simulink model "RBCM_Model"  (R2024b)
settings: Solver=FixedStepAuto  StartTime=0.0  StopTime=10.0  RelTol=1e-3
PreLoadFcn:
  | % NXP_MBDT_S32K3 callback: DO NOT REMOVE
  | mbd_s32k3.common.nxp.model_callbacks.preLoadFcn();
PostLoadFcn:
  | % NXP_MBDT_S32K3 callback: DO NOT REMOVE
  | mbd_s32k3.common.nxp.model_callbacks.postLoadFcn();
InitFcn:
  | % NXP_MBDT_S32K3 callback: DO NOT REMOVE
  | mbd_s32k3.common.nxp.model_callbacks.initFcn();
undefined symbols (not defined in the file or in its folder): AccuFanPwr_hHsd3ch2, BspdPwr_lHsd1ch2, BuzzerPwr_lHsd3ch3, DevicePwr_12v_lHsd1ch1, DevicePwr_hHsd1ch2, DrsPwr_8v_lHsd3ch1, hHsd_Diagnose_AdcBuffer, ILPwr_hHsd1ch1, lHsd_Diagnose_AdcBuffer, LoggerPwr_lHsd1ch3, PumpFan1_hHsd4ch1, PumpFan2_hHsd4ch2, PumpPwr_hHsd3ch1, RGBLED0state, TaillightPwr_lHsd3ch4, TempSensorPwr_lHsd1ch4
libraries: mbd_s32k3_io_library x127, simulink x48, canmsglib x8, mbd_s32k3_communication_library x7, mbd_s32k3_isr_library x6, mbd_s32k3_cdd_library x3, mbd_s32k3_utility_library x1
(part 4 of 10)

== system RBCM_Model/Subsystem1 ==
  note: 每通道采样次数|从1开始
  note: 最后一个指向|从1开始
  Trigger : TriggerPort  TriggerType=function-call  VariantControl=Variant
  Adc1 : mbd_s32k3_io_library/Adc  api_func=Adc_GetStreamLastPointer  hw_unit=AdcHwUnit_0  group=Adc0Group_1  channel=hpHSD2_IS_PTD20  threshold_control=AdcThresholdControl_0  power_state=ADC_FULL_POWER  ctu_trigger=AdcHwTrigger_0  ctu_fifo_idx=0  text=<binary blob, 41534 chars, not shown>
      settings: SourceProductName=IO Blocks
  Data Store Write1 : DataStoreWrite  DataStoreName=hHsd_Diagnose_AdcBuffer  DataStoreElements=hHsd_Diagnose_AdcBuffer(2)#hHsd_Diagnose_AdcBuffer(4)#hHsd_Diagnose_AdcBuffer(5)  IndexOptions=Index vector (dialog)  Indices=1  OutputSizes=1
  Data Store Write2 : DataStoreWrite  DataStoreName=lHsd_Diagnose_AdcBuffer  DataStoreElements=lHsd_Diagnose_AdcBuffer(1)#lHsd_Diagnose_AdcBuffer(2)#lHsd_Diagnose_AdcBuffer(5)  IndexOptions=Index vector (dialog)  Indices=1  OutputSizes=1
  Selector1 : Selector  IndexOptions=Index vector (dialog)  Indices=3  OutputSizes=1
  Selector2 : Selector  IndexOptions=Index vector (dialog)  Indices=4  OutputSizes=1
  Selector3 : Selector  IndexOptions=Index vector (dialog)  Indices=5  OutputSizes=1
  Selector4 : Selector  IndexOptions=Index vector (dialog)  Indices=1  OutputSizes=1
  Selector5 : Selector  IndexOptions=Index vector (dialog)  Indices=2  OutputSizes=1
  Selector6 : Selector  IndexOptions=Index vector (dialog)  Indices=6  OutputSizes=1
  Signal Specification : SignalSpecification  OutDataTypeStr=uint16  Dimensions=6
  Terminator1 : Terminator
  Terminator2 : Terminator
  wires:
  Adc1/3 -> Signal Specification/1
  Signal Specification/1 -> Selector6/1, Selector3/1, Selector2/1, Selector1/1, Selector5/1, Selector4/1
  Adc1/1 -> Terminator1/1
  Adc1/2 -> Terminator2/1
  Selector4/1 -> Data Store Write2/1
  Selector5/1 -> Data Store Write2/2
  Selector1/1 -> Data Store Write2/3
  Selector2/1 -> Data Store Write1/1
  Selector3/1 -> Data Store Write1/2
  Selector6/1 -> Data Store Write1/3

== system RBCM_Model/Subsystem10 ==
  In1 : Inport
  Bus Creator : BusCreator  Inputs=1
  Bus Selector : BusSelector  OutputSignals=signal1,signal1,signal1
  Selector1 : Selector  InputPortWidth=41  IndexOptions=Index vector (dialog)  Indices=[20 21 22 23 32 33 34 35]  OutputSizes=1
  Selector2 : Selector  InputPortWidth=41  IndexOptions=Index vector (dialog)  Indices=[16 17 18 19 28 29 30 31]  OutputSizes=1
  Selector3 : Selector  InputPortWidth=41  IndexOptions=Index vector (dialog)  Indices=[12 13 14 15 24 25 26 27]  OutputSizes=1
  Out1 : Outport
  Out2 : Outport  Port=2
  Out3 : Outport  Port=3
  wires:
  In1/1 -> Bus Creator/1
  Bus Selector/2 -> Selector2/1  "<signal1>"
  Selector2/1 -> Out2/1
  Selector3/1 -> Out1/1
  Selector1/1 -> Out3/1
  Bus Selector/3 -> Selector1/1  "<signal1>"
  Bus Selector/1 -> Selector3/1  "<signal1>"
  Bus Creator/1 -> Bus Selector/1

== system RBCM_Model/Subsystem11 ==
  note: 最后一个指向|从1开始
  note: 每通道采样次数|从1开始
  Trigger : TriggerPort  TriggerType=function-call  VariantControl=Variant
  Adc1 : mbd_s32k3_io_library/Adc  api_func=Adc_GetStreamLastPointer  hw_unit=AdcHwUnit_0  group=Adc1Group_1  channel=hpHSD2_IS_PTD20  threshold_control=AdcThresholdControl_0  power_state=ADC_FULL_POWER  ctu_trigger=AdcHwTrigger_0  ctu_fifo_idx=0  text=<binary blob, 41534 chars, not shown>
      settings: SourceProductName=IO Blocks
  Data Store Write : DataStoreWrite  DataStoreName=Temp_AdcBuffer  IndexOptions=Index vector (dialog)  Indices=1  OutputSizes=1
  Data Store Write1 : DataStoreWrite  DataStoreName=hHsd_Diagnose_AdcBuffer  DataStoreElements=hHsd_Diagnose_AdcBuffer(6)  IndexOptions=Index vector (dialog)  Indices=1  OutputSizes=1
  Data Store Write2 : DataStoreWrite  DataStoreName=lHsd_Diagnose_AdcBuffer  DataStoreElements=lHsd_Diagnose_AdcBuffer(4)  IndexOptions=Index vector (dialog)  Indices=1  OutputSizes=1
  Selector1 : Selector  IndexOptions=Index vector (dialog)  Indices=3  OutputSizes=1
  Selector4 : Selector  IndexOptions=Index vector (dialog)  Indices=1  OutputSizes=1
  Selector5 : Selector  IndexOptions=Index vector (dialog)  Indices=2  OutputSizes=1
  Signal Specification : SignalSpecification  OutDataTypeStr=uint16  Dimensions=3
  Terminator1 : Terminator
  Terminator2 : Terminator
  wires:
  Selector4/1 -> Data Store Write/1
  Adc1/2 -> Terminator2/1
  Adc1/1 -> Terminator1/1
  Signal Specification/1 -> Selector4/1, Selector5/1, Selector1/1
  Adc1/3 -> Signal Specification/1
  Selector5/1 -> Data Store Write2/1
  Selector1/1 -> Data Store Write1/1

== system RBCM_Model/Subsystem12 ==
  note: 每通道采样次数|从1开始
  note: 最后一个指向|从1开始
  Trigger : TriggerPort  TriggerType=function-call  VariantControl=Variant
  Adc1 : mbd_s32k3_io_library/Adc  api_func=Adc_GetStreamLastPointer  hw_unit=AdcHwUnit_0  group=Adc2Group_1  channel=hpHSD2_IS_PTD20  threshold_control=AdcThresholdControl_0  power_state=ADC_FULL_POWER  ctu_trigger=AdcHwTrigger_0  ctu_fifo_idx=0  text=<binary blob, 41534 chars, not shown>
      settings: SourceProductName=IO Blocks
  Data Store Write : DataStoreWrite  DataStoreName=hHsd_Diagnose_AdcBuffer  DataStoreElements=hHsd_Diagnose_AdcBuffer(1)#hHsd_Diagnose_AdcBuffer(3)  IndexOptions=Index vector (dialog)  Indices=1  OutputSizes=1
  Data Store Write1 : DataStoreWrite  DataStoreName=Bats_Monitor_AdcBuffer  DataStoreElements=Bats_Monitor_AdcBuffer(1)#Bats_Monitor_AdcBuffer(2)  IndexOptions=Index vector (dialog)  Indices=1  OutputSizes=1
  Data Store Write2 : DataStoreWrite  DataStoreName=lHsd_Diagnose_AdcBuffer  DataStoreElements=lHsd_Diagnose_AdcBuffer(3)  IndexOptions=Index vector (dialog)  Indices=1  OutputSizes=1
  Selector1 : Selector  IndexOptions=Index vector (dialog)  Indices=3  OutputSizes=1
  Selector2 : Selector  IndexOptions=Index vector (dialog)  Indices=4  OutputSizes=1
  Selector3 : Selector  IndexOptions=Index vector (dialog)  Indices=5  OutputSizes=1
  Selector4 : Selector  IndexOptions=Index vector (dialog)  Indices=1  OutputSizes=1
  Selector5 : Selector  IndexOptions=Index vector (dialog)  Indices=2  OutputSizes=1
  Signal Specification : SignalSpecification  OutDataTypeStr=uint16  Dimensions=5
  Terminator1 : Terminator
  Terminator2 : Terminator
  wires:
  Adc1/3 -> Signal Specification/1
  Signal Specification/1 -> Selector3/1, Selector2/1, Selector1/1, Selector5/1, Selector4/1
  Adc1/1 -> Terminator1/1
  Adc1/2 -> Terminator2/1
  Selector4/1 -> Data Store Write2/1
  Selector5/1 -> Data Store Write/1
  Selector1/1 -> Data Store Write/2
  Selector2/1 -> Data Store Write1/1
  Selector3/1 -> Data Store Write1/2

== system RBCM_Model/Subsystem13 ==
  In1 : Inport
  In2 : Inport  Port=2
  HsdDriveCommands : Merge
  If : If
  Subsystem : Subsystem
  Subsystem13 : Subsystem
  y1 : Outport
  wires:
  If/1 -> Subsystem13/Action
  If/2 -> Subsystem/Action
  In1/1 -> If/1
  HsdDriveCommands/1 -> y1/1
  Subsystem/1(y) -> HsdDriveCommands/1
  Subsystem13/1(Out1) -> HsdDriveCommands/2
  In2/1 -> Subsystem13/1(In1)

== system RBCM_Model/Subsystem2 ==
  note: 这一套输出经电脑测试可以正常连接服务器并MQTT通信
  output : Inport
  Add '\r\n'2 : MATLAB Function  TreatAsAtomicUnit=on
  Constant : Constant  Commented=on  Value=32
  Constant3 : Constant  Commented=on  Value=25
  MATLAB Function : MATLAB Function  Commented=on  TreatAsAtomicUnit=on
  String to ASCII : StringToASCII  OutputVectorSize=1024
  String to ASCII1 : StringToASCII  Commented=on  OutputVectorSize=3
  String to ASCII2 : StringToASCII  Commented=on  OutputVectorSize=3
  Terminator1 : Terminator
  To String : ToString  Commented=on
  To String1 : ToString  Commented=on
  Uart : mbd_s32k3_cdd_library/Uart  api_func=Uart_AsyncSend  channel=UartChannel_0  baudrate=UART_BAUDRATE_1200  transfer_type=UART_SEND  timeout=0  text=<binary blob, 5810 chars, not shown>
      settings: SourceProductName=CDD Blocks
  wires:
  Uart/1 -> Terminator1/1
  Add '\r\n'2/1(y) -> Uart/1
  output/1 -> String to ASCII/1
  String to ASCII/1 -> Add '\r\n'2/1(u)
  Constant/1 -> To String/1
  To String1/1 -> String to ASCII2/1
  String to ASCII1/1 -> MATLAB Function/1(temp1)
  String to ASCII2/1 -> MATLAB Function/2(temp2)
  Constant3/1 -> To String1/1
  To String/1 -> String to ASCII1/1

== system RBCM_Model/Subsystem5 ==
  In1 : Inport
  In2 : Inport  Port=2
  If : If
  Merge : Merge
  Subsystem : Subsystem
  Subsystem13 : Subsystem
  y1 : Outport
  wires:
  If/1 -> Subsystem13/Action
  If/2 -> Subsystem/Action
  In1/1 -> If/1
  Merge/1 -> y1/1
  Subsystem/1(y) -> Merge/1
  Subsystem13/1(Out1) -> Merge/2
  In2/1 -> Subsystem13/1(In1)

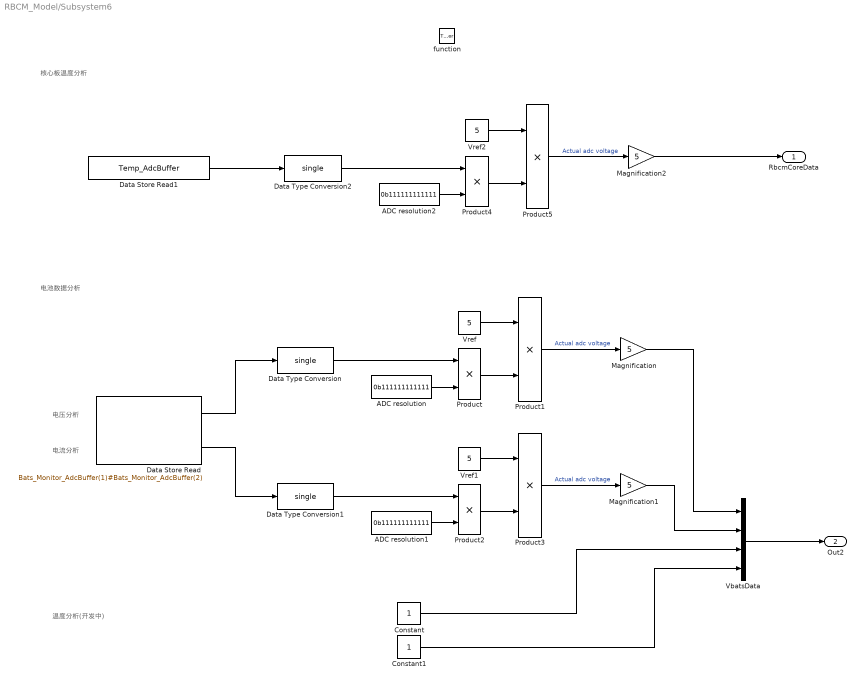
== system RBCM_Model/Subsystem6 ==
  note: 电压分析
  note: 电流分析
  note: 温度分析(开发中)
  note: 核心板温度分析
  note: 电池数据分析
  function : TriggerPort  TriggerType=function-call  VariantControl=Variant
  ADC resolution : Constant  Value=0b111111111111  OutDataTypeStr=uint16
  ADC resolution1 : Constant  Value=0b111111111111  OutDataTypeStr=uint16
  ADC resolution2 : Constant  Value=0b111111111111  OutDataTypeStr=uint16
  Constant : Constant  OutDataTypeStr=uint16
  Constant1 : Constant  OutDataTypeStr=uint16
  Data Store Read : DataStoreRead  DataStoreName=Bats_Monitor_AdcBuffer  DataStoreElements=Bats_Monitor_AdcBuffer(1)#Bats_Monitor_AdcBuffer(2)  IndexOptions=Index vector (dialog)  Indices=1  OutputSizes=1
  Data Store Read1 : DataStoreRead  DataStoreName=Temp_AdcBuffer  IndexOptions=Index vector (dialog)  Indices=1  OutputSizes=1
  Data Type Conversion : DataTypeConversion  OutDataTypeStr=single  SaturateOnIntegerOverflow=off  RndMeth=Floor
  Data Type Conversion1 : DataTypeConversion  OutDataTypeStr=single  SaturateOnIntegerOverflow=off  RndMeth=Floor
  Data Type Conversion2 : DataTypeConversion  OutDataTypeStr=single  SaturateOnIntegerOverflow=off  RndMeth=Floor
  Magnification : Gain  Gain=5  OutDataTypeStr=uint16
  Magnification1 : Gain  Gain=5  OutDataTypeStr=uint16
  Magnification2 : Gain  Gain=5  OutDataTypeStr=uint16
  Product{,1..5} (6 alike) : Product  OutDataTypeStr=single
  VbatsData : BusCreator  Inputs=4  OutDataTypeStr=Bus: Bus_Vbats_Data  NonVirtualBus=on
      settings: InheritFromInputs=off
  Vref : Constant  Value=5  OutDataTypeStr=uint8
  Vref1 : Constant  Value=5  OutDataTypeStr=uint8
  Vref2 : Constant  Value=5  OutDataTypeStr=uint8
  RbcmCoreData : Outport
  Out2 : Outport  Port=2  OutDataTypeStr=Bus: Bus_Vbats_Data
  wires:
  Data Store Read/1 -> Data Type Conversion/1
  Data Type Conversion/1 -> Product/1
  Product/1 -> Product1/2
  Vref/1 -> Product1/1
  ADC resolution/1 -> Product/2
  Product1/1 -> Magnification/1  "Actual adc voltage"
  Magnification/1 -> VbatsData/1
  Product3/1 -> Magnification1/1  "Actual adc voltage"
  ADC resolution1/1 -> Product2/2
  Vref1/1 -> Product3/1
  Product2/1 -> Product3/2
  Data Type Conversion1/1 -> Product2/1
  Magnification1/1 -> VbatsData/2
  Data Store Read/2 -> Data Type Conversion1/1
  VbatsData/1 -> Out2/1
  Constant/1 -> VbatsData/3
  Constant1/1 -> VbatsData/4
  Data Type Conversion2/1 -> Product4/1
  Product4/1 -> Product5/2
  Product5/1 -> Magnification2/1  "Actual adc voltage"
  Vref2/1 -> Product5/1
  ADC resolution2/1 -> Product4/2
  Data Store Read1/1 -> Data Type Conversion2/1
  Magnification2/1 -> RbcmCoreData/1

== system RBCM_Model/Subsystem7 ==
  function : TriggerPort  TriggerType=function-call  VariantControl=Variant
  Chart2 : Stateflow chart  TreatAsAtomicUnit=on
  Data Store Read : DataStoreRead  DataStoreName=RGBLED0state  DataStoreElements=RGBLED0state(1)#RGBLED0state(2)#RGBLED0state(3)  IndexOptions=Index vector (dialog)  Indices=1  OutputSizes=1
  Data Store Write : DataStoreWrite  DataStoreName=RGBLED0state  DataStoreElements=RGBLED0state(3)  IndexOptions=Index vector (dialog)  Indices=1  OutputSizes=1
  Data Type Conversion{1..3,13} (4 alike) : DataTypeConversion  OutDataTypeStr=uint8  SaturateOnIntegerOverflow=off  RndMeth=Floor
  Dio : mbd_s32k3_io_library/Dio  api_func=Dio_WriteChannel  channel=RGBLED0_BLUE  channel_group=No channel groups configured  port=PTB_H  gpioSim=on  text=<binary blob, 15399 chars, not shown>
      settings: SourceProductName=IO Blocks
  Dio1 : mbd_s32k3_io_library/Dio  api_func=Dio_WriteChannel  channel=RGBLED0_GREEN  channel_group=No channel groups configured  port=PTB_H  gpioSim=on  text=<binary blob, 15399 chars, not shown>
      settings: SourceProductName=IO Blocks
  Dio2 : mbd_s32k3_io_library/Dio  api_func=Dio_WriteChannel  channel=LED_PTB14  channel_group=No channel groups configured  port=PTB_H  gpioSim=on  text=<binary blob, 15399 chars, not shown>
      settings: SourceProductName=IO Blocks
  Dio3 : mbd_s32k3_io_library/Dio  api_func=Dio_WriteChannel  channel=RGBLED0_BLUE  channel_group=No channel groups configured  port=PTB_H  gpioSim=on  text=<binary blob, 15399 chars, not shown>
      settings: SourceProductName=IO Blocks
  wires:
  Data Type Conversion13/1 -> Dio/1
  Data Type Conversion1/1 -> Dio1/1
  Data Store Read/2 -> Data Type Conversion1/1
  Data Store Read/1 -> Data Type Conversion13/1
  Data Type Conversion2/1 -> Dio3/1, Dio2/1
  Data Store Read/3 -> Data Type Conversion2/1
  Chart2/1(" A") -> Data Type Conversion3/1
  Data Type Conversion3/1 -> Data Store Write/1

== system RBCM_Model/Subsystem8 ==
  note: GPIO＋PWM配合控制设备
      | DRS控制 PTD12 CH2 E33调频:333Hz-999Hz
  In5 : Inport
  function : TriggerPort  TriggerType=function-call  VariantControl=Variant
  Data Type Conversion4 : DataTypeConversion  SaturateOnIntegerOverflow=off  RndMeth=Floor
  Pwm : mbd_s32k3_io_library/Pwm  api_func=Pwm_SetDutyCycle  channel=PwmChannel_0  notification=PWM_RISING_EDGE  moduleId=PWM_EMIOS_INSTANCE_0  prescalerType=PWM_PRIMARY_PRESCALER  text=|
      | CommonPublishedInformation - CommonPublishedInformation Pwm 
      | CommonPublishedInformation/ArReleaseMajorVersion - 4 
      | CommonPublishedInformation/ArReleaseMinorVersion - 4 
      | CommonPublishedInformation/ArReleaseRevisionVersion - 0 
      | CommonPublishedInformation/ModuleId - 121 
      | CommonPublishedInformation/SwMajorVersion - 2 
      | CommonPublishedInformation/SwMinorVersion - 0 
      | CommonPublishedInformation/SwPatchVersion - 0 
      | CommonPublishedInformation/VendorId - 43 
      | IMPLEMENTATION-CONFIG-VARIANT - VARIANT-POST-BUILD 
      | POST_BUILD_VARIANT_USED - true 
      | PwmChannel - PwmChannel_0 PwmChannel_1 PwmChannel_2 PwmChannel_3 PwmChannel_4 PwmChannel_5 PwmChannel_6 PwmChannel_7 PwmChannel_8 
      | PwmChannel_0/Index - 0 
      | PwmChannel_0/PwmChannelId - 0 
      | PwmChannel_0/PwmDutycycleDefault - 2048 
      | PwmChannel_0/PwmHwChannel - /Pwm/Pwm/PwmChannelConfigSet/PwmEmios_0/PwmEmiosChannels_9 
      | PwmChannel_0/PwmIdleState - PWM_LOW 
      | PwmChannel_0/PwmMcuClockReferencePoint - /Mcu/Mcu/McuModuleConfiguration/McuClockSettingConfig_0/CORE_CLK 
      | PwmChannel_0/PwmNotification - PwmChannel_0_Callback 
      | PwmChannel_0/PwmPeriodDefault - 16000.0 
      | PwmChannel_0/PwmPeriodInTicks - true 
      | PwmChannel_0/PwmPolarity - PWM_HIGH 
      | PwmChannel_1/Index - 1 
      | PwmChannel_1/PwmChannelId - 1 
      | PwmChannel_1/PwmDutycycleDefault - 2048 
      | PwmChannel_1/PwmHwChannel - /Pwm/Pwm/PwmChannelConfigSet/PwmEmios_0/PwmEmiosChannels_17 
      | PwmChannel_1/PwmIdleState - PWM_LOW 
      | PwmChannel_1/PwmMcuClockReferencePoint - /Mcu/Mcu/McuModuleConfiguration/McuClockSettingConfig_0/CORE_CLK 
      | PwmChannel_1/PwmNotification - PwmChannel_1_Callback 
      | PwmChannel_1/PwmPeriodDefault - 16000.0 
      | PwmChannel_1/PwmPeriodInTicks - true 
      | PwmChannel_1/PwmPolarity - PWM_HIGH 
      | PwmChannel_2/Index - 2 
      | PwmChannel_2/PwmChannelId - 2 
      | PwmChannel_2/PwmDutycycleDefault - 0 
      | PwmChannel_2/PwmHwChannel - /Pwm/Pwm/PwmChannelConfigSet/PwmEmios_1/PwmEmiosChannels_19 
      | PwmChannel_2/PwmIdleState - PWM_LOW 
      | PwmChannel_2/PwmMcuClockReferencePoint - /Mcu/Mcu/McuModuleConfiguration/McuClockSettingConfig_0/CORE_CLK 
      | PwmChannel_2/PwmNotification - PwmChannel_2_Callback 
      | PwmChannel_2/PwmPeriodDefault - 16000.0 
      | PwmChannel_2/PwmPeriodInTicks - true 
      | PwmChannel_2/PwmPolarity - PWM_HIGH 
      | PwmChannel_3/Index - 3 
      | PwmChannel_3/PwmChannelId - 3 
      | PwmChannel_3/PwmDutycycleDefault - 0 
      | PwmChannel_3/PwmHwChannel - /Pwm/Pwm/PwmChannelConfigSet/PwmEmios_1/PwmEmiosChannels_20 
      | PwmChannel_3/PwmIdleState - PWM_LOW 
      | PwmChannel_3/PwmMcuClockReferencePoint - /Mcu/Mcu/McuModuleConfiguration/McuClockSettingConfig_0/CORE_CLK 
      | PwmChannel_3/PwmNotification - PwmChannel_3_Callback 
      | PwmChannel_3/PwmPeriodDefault - 16000.0 
      | PwmChannel_3/PwmPeriodInTicks - true 
      | PwmChannel_3/PwmPolarity - PWM_HIGH 
      | PwmChannel_4/Index - 4 
      | PwmChannel_4/PwmChannelId - 4 
      | PwmChannel_4/PwmDutycycleDefault - 0 
      | PwmChannel_4/PwmHwChannel - /Pwm/Pwm/PwmChannelConfigSet/PwmEmios_1/PwmEmiosChannels_0 
      | PwmChannel_4/PwmIdleState - PWM_LOW 
      | PwmChannel_4/PwmMcuClockReferencePoint - /Mcu/Mcu/McuModuleConfiguration/McuClockSettingConfig_0/CORE_CLK 
      | PwmChannel_4/PwmNotification - PwmChannel_4_Callback 
      | PwmChannel_4/PwmPeriodDefault - 16000.0 
      | PwmChannel_4/PwmPeriodInTicks - true 
      | PwmChannel_4/PwmPolarity - PWM_HIGH 
      | PwmChannel_5/Index - 5 
      | PwmChannel_5/PwmChannelId - 5 
      | PwmChannel_5/PwmDutycycleDefault - 0 
      | PwmChannel_5/PwmHwChannel - /Pwm/Pwm/PwmChannelConfigSet/PwmEmios_1/PwmEmiosChannels_1 
      | PwmChannel_5/PwmIdleState - PWM_LOW 
      | PwmChannel_5/PwmMcuClockReferencePoint - /Mcu/Mcu/McuModuleConfiguration/McuClockSettingConfig_0/CORE_CLK 
      | PwmChannel_5/PwmNotification - PwmChannel_5_Callback 
      | PwmChannel_5/PwmPeriodDefault - 16000.0 
      | PwmChannel_5/PwmPeriodInTicks - true 
      | PwmChannel_5/PwmPolarity - PWM_HIGH 
      | PwmChannel_6/Index - 6 
      | PwmChannel_6/PwmChannelId - 6 
      | PwmChannel_6/PwmDutycycleDefault - 0 
      | PwmChannel_6/PwmHwChannel - /Pwm/Pwm/PwmChannelConfigSet/PwmEmios_1/PwmEmiosChannels_21 
      | PwmChannel_6/PwmIdleState - PWM_LOW 
      | PwmChannel_6/PwmMcuClockReferencePoint - /Mcu/Mcu/McuModuleConfiguration/McuClockSettingConfig_0/CORE_CLK 
      | PwmChannel_6/PwmNotification - PwmChannel_6_Callback 
      | PwmChannel_6/PwmPeriodDefault - 16000.0 
      | PwmChannel_6/PwmPeriodInTicks - true 
      | PwmChannel_6/PwmPolarity - PWM_HIGH 
      | PwmChannel_7/Index - 7 
      | PwmChannel_7/PwmChannelId - 7 
      | PwmChannel_7/PwmDutycycleDefault - 0 
      | PwmChannel_7/PwmHwChannel - /Pwm/Pwm/PwmChannelConfigSet/PwmEmios_1/PwmEmiosChannels_22 
      | PwmChannel_7/PwmIdleState - PWM_LOW 
      | PwmChannel_7/PwmMcuClockReferencePoint - /Mcu/Mcu/McuModuleConfiguration/McuClockSettingConfig_0/CORE_CLK 
      | PwmChannel_7/PwmNotification - PwmChannel_7_Callback 
      | PwmChannel_7/PwmPeriodDefault - 16000.0 
      | PwmChannel_7/PwmPeriodInTicks - true 
      | PwmChannel_7/PwmPolarity - PWM_HIGH 
      | PwmChannel_8/Index - 8 
      | PwmChannel_8/PwmChannelId - 8 
      | PwmChannel_8/PwmDutycycleDefault - 0 
      | PwmChannel_8/PwmHwChannel - /Pwm/Pwm/PwmChannelConfigSet/PwmEmios_2/PwmEmiosChannels_7 
      | PwmChannel_8/PwmIdleState - PWM_LOW 
      | PwmChannel_8/PwmMcuClockReferencePoint - /Mcu/Mcu/McuModuleConfiguration/McuClockSettingConfig_0/CORE_CLK 
      | PwmChannel_8/PwmNotification - PwmChannel_8_Callback 
      | PwmChannel_8/PwmPeriodDefault - 40000 
      | PwmChannel_8/PwmPeriodInTicks - true 
      | PwmChannel_8/PwmPolarity - PWM_HIGH 
      | PwmConfigurationOfOptApiServices - PwmConfigurationOfOptApiServices 
      | PwmConfigurationOfOptApiServices/PwmDeInitApi - true 
      | PwmConfigurationOfOptApiServices/PwmEmiosFastUpdateApi - true 
      | PwmConfigurationOfOptApiServices/PwmEnableMaskOutputs - false 
      | PwmConfigurationOfOptApiServices/PwmGetChannelStateApi - true 
      | PwmConfigurationOfOptApiServices/PwmGetOutputState - true 
      | PwmConfigurationOfOptApiServices/PwmSetChannelDeadTime - true 
      | PwmConfigurationOfOptApiServices/PwmSetChannelOutputApi - true 
      | PwmConfigurationOfOptApiServices/PwmSetCounterBusApi - true 
      | PwmConfigurationOfOptApiServices/PwmSetDutyCycle - true 
      | PwmConfigurationOfOptApiServices/PwmSetDutyCycle_NoUpdate - false 
      | PwmConfigurationOfOptApiServices/PwmSetDutyPhaseShift - false 
      | PwmConfigurationOfOptApiServices/PwmSetOutputToIdle - true 
      | PwmConfigurationOfOptApiServices/PwmSetPeriodAndDuty - true 
      | PwmConfigurationOfOptApiServices/PwmSetPeriodAndDuty_NoUpdate - false 
      | PwmConfigurationOfOptApiServices/PwmSetTriggerDelayApi - true 
      | PwmConfigurationOfOptApiServices/PwmVersionInfoApi - true 
      | PwmEmios - PwmEmios_0 PwmEmios_1 PwmEmios_2 
      | PwmEmios_0/Index - 0 
      | PwmEmios_0/PwmEmiosChannels - PwmEmiosChannels_17 PwmEmiosChannels_9 
      | PwmEmios_0/PwmEmiosChannels_17/EmiosChCounterBus - EMIOS_PWM_IP_BUS_A 
      | PwmEmios_0/PwmEmiosChannels_17/EmiosChDeadtime - 0 
      | PwmEmios_0/PwmEmiosChannels_17/EmiosChFlagGeneration - Trailing_Edge 
      | PwmEmios_0/PwmEmiosChannels_17/EmiosChFreeze - false 
      | PwmEmios_0/PwmEmiosChannels_17/EmiosChId - CH_17 
      | PwmEmios_0/PwmEmiosChannels_17/EmiosChInterrupt - EMIOS_PWM_IP_INTERRUPT_REQUEST 
      | PwmEmios_0/PwmEmiosChannels_17/EmiosChMode - EMIOS_PWM_IP_MODE_OPWMB 
      | PwmEmios_0/PwmEmiosChannels_17/EmiosChOutputDisable - EMIOS_PWM_IP_OUTPUT_DISABLE_NONE 
      | PwmEmios_0/PwmEmiosChannels_17/EmiosChPhaseShift - 0 
      | PwmEmios_0/PwmEmiosChannels_17/EmiosChPrescaler - EMIOS_PWM_IP_CLOCK_DIV_2 
      | PwmEmios_0/PwmEmiosChannels_17/EmiosChPrescalerAlternate - EMIOS_PWM_IP_CLOCK_DIV_1 
      | PwmEmios_0/PwmEmiosChannels_17/EmiosChPrescalerSource - EMIOS_PWM_IP_PS_SRC_MODULE_CLOCK 
      | PwmEmios_0/PwmEmiosChannels_17/EmiosChTrigger - 0 
      | PwmEmios_0/PwmEmiosChannels_17/Index - 1 
      | PwmEmios_0/PwmEmiosChannels_17/PwmEmiosBusRef - /Mcl/Mcl/MclConfig/EmiosCommon_0/EmiosMclMasterBus_0 
      | PwmEmios_0/PwmEmiosChannels_9/EmiosChCounterBus - EMIOS_PWM_IP_BUS_A 
      | PwmEmios_0/PwmEmiosChannels_9/EmiosChDeadtime - 0 
      | PwmEmios_0/PwmEmiosChannels_9/EmiosChFlagGeneration - Trailing_Edge 
      | PwmEmios_0/PwmEmiosChannels_9/EmiosChFreeze - false 
      | PwmEmios_0/PwmEmiosChannels_9/EmiosChId - CH_9 
      | PwmEmios_0/PwmEmiosChannels_9/EmiosChInterrupt - EMIOS_PWM_IP_INTERRUPT_REQUEST 
      | PwmEmios_0/PwmEmiosChannels_9/EmiosChMode - EMIOS_PWM_IP_MODE_OPWMB 
      | PwmEmios_0/PwmEmiosChannels_9/EmiosChOutputDisable - EMIOS_PWM_IP_OUTPUT_DISABLE_NONE 
      | PwmEmios_0/PwmEmiosChannels_9/EmiosChPhaseShift - 0 
      | PwmEmios_0/PwmEmiosChannels_9/EmiosChPrescaler - EMIOS_PWM_IP_CLOCK_DIV_1 
      | PwmEmios_0/PwmEmiosChannels_9/EmiosChPrescalerAlternate - EMIOS_PWM_IP_CLOCK_DIV_1 
      | PwmEmios_0/PwmEmiosChannels_9/EmiosChPrescalerSource - EMIOS_PWM_IP_PS_SRC_MODULE_CLOCK 
      | PwmEmios_0/PwmEmiosChannels_9/EmiosChTrigger - 0 
      | PwmEmios_0/PwmEmiosChannels_9/Index - 0 
      | PwmEmios_0/PwmEmiosChannels_9/PwmEmiosBusRef - /Mcl/Mcl/MclConfig/EmiosCommon_0/EmiosMclMasterBus_0 
      | PwmEmios_0/PwmHwInstance - Emios_0 
      | PwmEmios_1/Index - 1 
      | PwmEmios_1/PwmEmiosChannels - PwmEmiosChannels_0 PwmEmiosChannels_1 PwmEmiosChannels_19 PwmEmiosChannels_20 PwmEmiosChannels_21 PwmEmiosChannels_22 
      | PwmEmios_1/PwmEmiosChannels_0/EmiosChCounterBus - EMIOS_PWM_IP_BUS_A 
      | PwmEmios_1/PwmEmiosChannels_0/EmiosChDeadtime - 0 
      | PwmEmios_1/PwmEmiosChannels_0/EmiosChFlagGeneration - Trailing_Edge 
      | PwmEmios_1/PwmEmiosChannels_0/EmiosChFreeze - false 
      | PwmEmios_1/PwmEmiosChannels_0/EmiosChId - CH_0 
      | PwmEmios_1/PwmEmiosChannels_0/EmiosChInterrupt - EMIOS_PWM_IP_INTERRUPT_REQUEST 
      | PwmEmios_1/PwmEmiosChannels_0/EmiosChMode - EMIOS_PWM_IP_MODE_OPWMB 
      | PwmEmios_1/PwmEmiosChannels_0/EmiosChOutputDisable - EMIOS_PWM_IP_OUTPUT_DISABLE_NONE 
      | PwmEmios_1/PwmEmiosChannels_0/EmiosChPhaseShift - 0 
      | PwmEmios_1/PwmEmiosChannels_0/EmiosChPrescaler - EMIOS_PWM_IP_CLOCK_DIV_1 
      | PwmEmios_1/PwmEmiosChannels_0/EmiosChPrescalerAlternate - EMIOS_PWM_IP_CLOCK_DIV_1 
      | PwmEmios_1/PwmEmiosChannels_0/EmiosChPrescalerSource - EMIOS_PWM_IP_PS_SRC_MODULE_CLOCK 
      | PwmEmios_1/PwmEmiosChannels_0/EmiosChTrigger - 0 
      | PwmEmios_1/PwmEmiosChannels_0/Index - 2 
      | PwmEmios_1/PwmEmiosChannels_0/PwmEmiosBusRef - /Mcl/Mcl/MclConfig/EmiosCommon_1/EmiosMclMasterBus_0 
      | PwmEmios_1/PwmEmiosChannels_1/EmiosChCounterBus - EMIOS_PWM_IP_BUS_A 
      | PwmEmios_1/PwmEmiosChannels_1/EmiosChDeadtime - 0 
      | PwmEmios_1/PwmEmiosChannels_1/EmiosChFlagGeneration - Trailing_Edge 
      | PwmEmios_1/PwmEmiosChannels_1/EmiosChFreeze - false 
      | PwmEmios_1/PwmEmiosChannels_1/EmiosChId - CH_1 
      | PwmEmios_1/PwmEmiosChannels_1/EmiosChInterrupt - EMIOS_PWM_IP_INTERRUPT_REQUEST 
      | PwmEmios_1/PwmEmiosChannels_1/EmiosChMode - EMIOS_PWM_IP_MODE_OPWMB 
      | PwmEmios_1/PwmEmiosChannels_1/EmiosChOutputDisable - EMIOS_PWM_IP_OUTPUT_DISABLE_NONE 
      | PwmEmios_1/PwmEmiosChannels_1/EmiosChPhaseShift - 0 
      | PwmEmios_1/PwmEmiosChannels_1/EmiosChPrescaler - EMIOS_PWM_IP_CLOCK_DIV_1 
      | PwmEmios_1/PwmEmiosChannels_1/EmiosChPrescalerAlternate - EMIOS_PWM_IP_CLOCK_DIV_1 
      | PwmEmios_1/PwmEmiosChannels_1/EmiosChPrescalerSource - EMIOS_PWM_IP_PS_SRC_MODULE_CLOCK 
      | PwmEmios_1/PwmEmiosChannels_1/EmiosChTrigger - 0 
      | PwmEmios_1/PwmEmiosChannels_1/Index - 3 
      | PwmEmios_1/PwmEmiosChannels_1/PwmEmiosBusRef - /Mcl/Mcl/MclConfig/EmiosCommon_1/EmiosMclMasterBus_0 
      | PwmEmios_1/PwmEmiosChannels_19/EmiosChCounterBus - EMIOS_PWM_IP_BUS_A 
      | PwmEmios_1/PwmEmiosChannels_19/EmiosChDeadtime - 0 
      | PwmEmios_1/PwmEmiosChannels_19/EmiosChFlagGeneration - Trailing_Edge 
      | PwmEmios_1/PwmEmiosChannels_19/EmiosChFreeze - false 
      | PwmEmios_1/PwmEmiosChannels_19/EmiosChId - CH_19 
      | PwmEmios_1/PwmEmiosChannels_19/EmiosChInterrupt - EMIOS_PWM_IP_INTERRUPT_REQUEST 
      | PwmEmios_1/PwmEmiosChannels_19/EmiosChMode - EMIOS_PWM_IP_MODE_OPWMB 
      | PwmEmios_1/PwmEmiosChannels_19/EmiosChOutputDisable - EMIOS_PWM_IP_OUTPUT_DISABLE_NONE 
      | PwmEmios_1/PwmEmiosChannels_19/EmiosChPhaseShift - 0 
      | PwmEmios_1/PwmEmiosChannels_19/EmiosChPrescaler - EMIOS_PWM_IP_CLOCK_DIV_1 
      | PwmEmios_1/PwmEmiosChannels_19/EmiosChPrescalerAlternate - EMIOS_PWM_IP_CLOCK_DIV_1 
      | PwmEmios_1/PwmEmiosChannels_19/EmiosChPrescalerSource - EMIOS_PWM_IP_PS_SRC_MODULE_CLOCK 
      | PwmEmios_1/PwmEmiosChannels_19/EmiosChTrigger - 0 
      | PwmEmios_1/PwmEmiosChannels_19/Index - 0 
      | PwmEmios_1/PwmEmiosChannels_19/PwmEmiosBusRef - /Mcl/Mcl/MclConfig/EmiosCommon_1/EmiosMclMasterBus_0 
      | PwmEmios_1/PwmEmiosChannels_20/EmiosChCounterBus - EMIOS_PWM_IP_BUS_A 
      | PwmEmios_1/PwmEmiosChannels_20/EmiosChDeadtime - 0 
      | PwmEmios_1/PwmEmiosChannels_20/EmiosChFlagGeneration - Trailing_Edge 
      | PwmEmios_1/PwmEmiosChannels_20/EmiosChFreeze - false 
      | PwmEmios_1/PwmEmiosChannels_20/EmiosChId - CH_20 
      | PwmEmios_1/PwmEmiosChannels_20/EmiosChInterrupt - EMIOS_PWM_IP_INTERRUPT_REQUEST 
      | PwmEmios_1/PwmEmiosChannels_20/EmiosChMode - EMIOS_PWM_IP_MODE_OPWMB 
      | PwmEmios_1/PwmEmiosChannels_20/EmiosChOutputDisable - EMIOS_PWM_IP_OUTPUT_DISABLE_NONE 
      | PwmEmios_1/PwmEmiosChannels_20/EmiosChPhaseShift - 0 
      | PwmEmios_1/PwmEmiosChannels_20/EmiosChPrescaler - EMIOS_PWM_IP_CLOCK_DIV_1 
      | PwmEmios_1/PwmEmiosChannels_20/EmiosChPrescalerAlternate - EMIOS_PWM_IP_CLOCK_DIV_1 
      | PwmEmios_1/PwmEmiosChannels_20/EmiosChPrescalerSource - EMIOS_PWM_IP_PS_SRC_MODULE_CLOCK 
      | PwmEmios_1/PwmEmiosChannels_20/EmiosChTrigger - 0 
      | PwmEmios_1/PwmEmiosChannels_20/Index - 1 
      | PwmEmios_1/PwmEmiosChannels_20/PwmEmiosBusRef - /Mcl/Mcl/MclConfig/EmiosCommon_1/EmiosMclMasterBus_0 
      | PwmEmios_1/PwmEmiosChannels_21/EmiosChCounterBus - EMIOS_PWM_IP_BUS_A 
      | PwmEmios_1/PwmEmiosChannels_21/EmiosChDeadtime - 0 
      | PwmEmios_1/PwmEmiosChannels_21/EmiosChFlagGeneration - Trailing_Edge 
      | PwmEmios_1/PwmEmiosChannels_21/EmiosChFreeze - false 
      | PwmEmios_1/PwmEmiosChannels_21/EmiosChId - CH_21 
      | PwmEmios_1/PwmEmiosChannels_21/EmiosChInterrupt - EMIOS_PWM_IP_INTERRUPT_REQUEST 
      | PwmEmios_1/PwmEmiosChannels_21/EmiosChMode - EMIOS_PWM_IP_MODE_OPWMB 
      | PwmEmios_1/PwmEmiosChannels_21/EmiosChOutputDisable - EMIOS_PWM_IP_OUTPUT_DISABLE_NONE 
      | PwmEmios_1/PwmEmiosChannels_21/EmiosChPhaseShift - 0 
      | PwmEmios_1/PwmEmiosChannels_21/EmiosChPrescaler - EMIOS_PWM_IP_CLOCK_DIV_1 
      | PwmEmios_1/PwmEmiosChannels_21/EmiosChPrescalerAlternate - EMIOS_PWM_IP_CLOCK_DIV_1 
      | PwmEmios_1/PwmEmiosChannels_21/EmiosChPrescalerSource - EMIOS_PWM_IP_PS_SRC_MODULE_CLOCK 
      | PwmEmios_1/PwmEmiosChannels_21/EmiosChTrigger - 0 
      | PwmEmios_1/PwmEmiosChannels_21/Index - 4 
      | PwmEmios_1/PwmEmiosChannels_21/PwmEmiosBusRef - /Mcl/Mcl/MclConfig/EmiosCommon_1/EmiosMclMasterBus_0 
      | PwmEmios_1/PwmEmiosChannels_22/EmiosChCounterBus - EMIOS_PWM_IP_BUS_A 
      | PwmEmios_1/PwmEmiosChannels_22/EmiosChDeadtime - 0 
      | PwmEmios_1/PwmEmiosChannels_22/EmiosChFlagGeneration - Trailing_Edge 
      | PwmEmios_1/PwmEmiosChannels_22/EmiosChFreeze - false 
      | PwmEmios_1/PwmEmiosChannels_22/EmiosChId - CH_22 
      | PwmEmios_1/PwmEmiosChannels_22/EmiosChInterrupt - EMIOS_PWM_IP_INTERRUPT_REQUEST 
      | PwmEmios_1/PwmEmiosChannels_22/EmiosChMode - EMIOS_PWM_IP_MODE_OPWMB 
      | PwmEmios_1/PwmEmiosChannels_22/EmiosChOutputDisable - EMIOS_PWM_IP_OUTPUT_DISABLE_NONE 
      | PwmEmios_1/PwmEmiosChannels_22/EmiosChPhaseShift - 0 
      | PwmEmios_1/PwmEmiosChannels_22/EmiosChPrescaler - EMIOS_PWM_IP_CLOCK_DIV_1 
      | PwmEmios_1/PwmEmiosChannels_22/EmiosChPrescalerAlternate - EMIOS_PWM_IP_CLOCK_DIV_1 
      | PwmEmios_1/PwmEmiosChannels_22/EmiosChPrescalerSource - EMIOS_PWM_IP_PS_SRC_MODULE_CLOCK 
      | PwmEmios_1/PwmEmiosChannels_22/EmiosChTrigger - 0 
      | PwmEmios_1/PwmEmiosChannels_22/Index - 5 
      | PwmEmios_1/PwmEmiosChannels_22/PwmEmiosBusRef - /Mcl/Mcl/MclConfig/EmiosCommon_1/EmiosMclMasterBus_0 
      | PwmEmios_1/PwmHwInstance - Emios_1 
      | PwmEmios_2/Index - 2 
      | PwmEmios_2/PwmEmiosChannels - PwmEmiosChannels_7 
      | PwmEmios_2/PwmEmiosChannels_7/EmiosChCounterBus - EMIOS_PWM_IP_BUS_A 
      | PwmEmios_2/PwmEmiosChannels_7/EmiosChDeadtime - 0 
      | PwmEmios_2/PwmEmiosChannels_7/EmiosChFlagGeneration - Trailing_Edge 
      | PwmEmios_2/PwmEmiosChannels_7/EmiosChFreeze - false 
      | PwmEmios_2/PwmEmiosChannels_7/EmiosChId - CH_7 
      | PwmEmios_2/PwmEmiosChannels_7/EmiosChInterrupt - EMIOS_PWM_IP_INTERRUPT_REQUEST 
      | PwmEmios_2/PwmEmiosChannels_7/EmiosChMode - EMIOS_PWM_IP_MODE_OPWMB 
      | PwmEmios_2/PwmEmiosChannels_7/EmiosChOutputDisable - EMIOS_PWM_IP_OUTPUT_DISABLE_NONE 
      | PwmEmios_2/PwmEmiosChannels_7/EmiosChPhaseShift - 0 
      | PwmEmios_2/PwmEmiosChannels_7/EmiosChPrescaler - EMIOS_PWM_IP_CLOCK_DIV_2 
      | PwmEmios_2/PwmEmiosChannels_7/EmiosChPrescalerAlternate - EMIOS_PWM_IP_CLOCK_DIV_2 
      | PwmEmios_2/PwmEmiosChannels_7/EmiosChPrescalerSource - EMIOS_PWM_IP_PS_SRC_MODULE_CLOCK 
      | PwmEmios_2/PwmEmiosChannels_7/EmiosChTrigger - 0 
      | PwmEmios_2/PwmEmiosChannels_7/Index - 0 
      | PwmEmios_2/PwmEmiosChannels_7/PwmEmiosBusRef - /Mcl/Mcl/MclConfig/EmiosCommon_2/EmiosMclMasterBus_0 
      | PwmEmios_2/PwmHwInstance - Emios_2 
      | PwmEtpu - PwmChannelConfigSet 
      | PwmGeneral - PwmGeneral 
      | PwmGeneral/PwmDevErrorDetect - true 
      | PwmGeneral/PwmDutycycleUpdatedEndperiod - false 
      | PwmGeneral/PwmEnableDualClockMode - false 
      | PwmGeneral/PwmEnableUserModeSupport - false 
      | PwmGeneral/PwmIndex - 0 
      | PwmGeneral/PwmMultiChannelSync - false 
      | PwmGeneral/PwmMultipartitionEnabled - false 
      | PwmGeneral/PwmNotificationSupported - true 
      | PwmGeneral/PwmPeriodUpdatedEndperiod - true
      settings: SourceProductName=IO Blocks
  wires:
  Data Type Conversion4/1 -> Pwm/1
  In5/1 -> Data Type Conversion4/1

== system RBCM_Model/Subsystem9 ==
  function : TriggerPort  VariantControl=Variant
  Add '\r\n' : MATLAB Function  TreatAsAtomicUnit=on
  Constant1 : Constant  Value=uint8('AT')  VectorParams1D=off
  Terminator1 : Terminator
  Uart1 : mbd_s32k3_cdd_library/Uart  api_func=Uart_AsyncSend  channel=UartChannel_0  baudrate=UART_BAUDRATE_1200  transfer_type=UART_SEND  timeout=0  text=<binary blob, 5810 chars, not shown>
      settings: SourceProductName=CDD Blocks
  wires:
  Add '\r\n'/1(y) -> Uart1/1
  Uart1/1 -> Terminator1/1
  Constant1/1 -> Add '\r\n'/1(u)

== system RBCM_Model/指令报文解码器 ==
  In1 : Inport  OutDataTypeStr=Bus: Bus_CAN_RX_MESSAG
  HsdDriveCommandsInit : Inport  Port=2  OutDataTypeStr=Bus: Bus_Hsd_Drive_Commands
  function : TriggerPort  TriggerType=function-call  VariantControl=Variant
  Chart1 : Stateflow chart  TreatAsAtomicUnit=on
  Data Store Write : DataStoreWrite  DataStoreName=RGBLED0state  DataStoreElements=RGBLED0state(2)  IndexOptions=Index vector (dialog)  Indices=1  OutputSizes=1
  Data Type Conversion13 : DataTypeConversion  OutDataTypeStr=uint8  SaturateOnIntegerOverflow=off  RndMeth=Floor
  Subsystem3 : Subsystem
  HsdDriveCommands : Outport
  DrsDriveCommand : Outport  Port=2
  VehicleData : Outport  Port=3
  wires:
  Chart1/1(" A") -> Data Type Conversion13/1
  Data Type Conversion13/1 -> Data Store Write/1
  Subsystem3/1(Out1) -> HsdDriveCommands/1
  HsdDriveCommandsInit/1 -> Subsystem3/2(In1)
  In1/1 -> Subsystem3/1(In2)
  Subsystem3/3(Out2) -> VehicleData/1
  Subsystem3/2(Out3) -> DrsDriveCommand/1

== system RBCM_Model/控制状态机 ==
  In2 : Inport
  function : TriggerPort  TriggerType=function-call  VariantControl=Variant  SampleTimeType=periodic  SampleTime=2
  4G通信控制状态机 : Stateflow chart  TreatAsAtomicUnit=on
  Chart1 : Stateflow chart  TreatAsAtomicUnit=on
  Constant : Constant  OutDataTypeStr=uint8
  Constant2 : Constant  OutDataTypeStr=uint8
  Data Store Write : DataStoreWrite  DataStoreName=init_finish_flag  IndexOptions=Index vector (dialog)  Indices=1  OutputSizes=1
  Data Type Conversion13 : DataTypeConversion  OutDataTypeStr=uint8  SaturateOnIntegerOverflow=off  RndMeth=Floor
  Dio : mbd_s32k3_io_library/Dio  api_func=Dio_WriteChannel  channel=RGBLED0_GREEN  channel_group=No channel groups configured  port=PTB_H  gpioSim=on  text=<binary blob, 15399 chars, not shown>
      settings: SourceProductName=IO Blocks
  output : Outport
  wires:
  Constant2/1 -> 4G通信控制状态机/3(timer)
  Constant/1 -> 4G通信控制状态机/2(enable)
  In2/1 -> 4G通信控制状态机/1(signal)
  Chart1/1(" A") -> Data Type Conversion13/1
  Data Type Conversion13/1 -> Dio/1
  4G通信控制状态机/2(endflag) -> Data Store Write/1
  4G通信控制状态机/1(output) -> output/1

== system RBCM_Model/无线调试模式管理子系统 ==
  function : TriggerPort  TriggerType=function-call  VariantControl=Variant
  Dio1 : mbd_s32k3_io_library/Dio  api_func=Dio_ReadChannel  channel=ESP32S3_EN  channel_group=No channel groups configured  port=PTB_H  gpioSim=off  text=<binary blob, 15399 chars, not shown>
      settings: SourceProductName=IO Blocks
  If : If  IfExpression=u1 == 0
  Subsystem : Subsystem
  Subsystem1 : Subsystem
  wires:
  If/2 -> Subsystem1/Action
  Dio1/1 -> If/1
  If/1 -> Subsystem/Action
